simulink model "dynamic_range_compression"  (R2020b)
settings: Solver=FixedStepAuto  StartTime=0.0  StopTime=stop_time  FixedStep=1  RelTol=1e-3
InitFcn:
  | test_FFT_to_gain_init
StopFcn:
  | test_FFT_to_gain_stop
values from neighbouring files (symbols this model uses):
  accum_delay = max(band_sizes)    [test_FFT_to_gain_init.m]
  accum_delay_memory_size = 2^accum_delay_memory    [test_FFT_to_gain_init.m]
  band_edges = [band_edges mirrored_band_edges]    [test_FFT_to_gain_init.m]
  buf_a = 65.*ones(num_bands,1)    [test_FFT_to_gain_init.m]    (also in test_db_ar_gaintable_init.m)
  buf_r = 65.*ones(num_bands,1)    [test_FFT_to_gain_init.m]    (also in test_db_ar_gaintable_init.m)
  delay_memory_size = 2^system_delay_memory    [test_FFT_to_gain_init.m]
  FFTsize = 256    [test_FFT_to_gain_init.m]    (also in test_db_ar_gaintable_init.m)
  gainapp_dp_memory = log2(num_bands) + 1    [test_FFT_to_gain_init.m]
  num_bands = 8    [test_FFT_to_gain_init.m]    (also in test_db_ar_gaintable_init.m = 2)
  num_bins = FFTsize/2 + 1    (= 129)    [test_FFT_to_gain_init.m]    (also in test_db_ar_gaintable_init.m)
  system_delay = 70    [calculate_gainapp_test_signals.m]    (also in test_FFT_to_gain_init.m = gain_delay + accum_delay)
  table_length = length(gtdata)    [test_FFT_to_gain_init.m]    (also in test_db_ar_gaintable_init.m)
  X_high = 93    [test_FFT_to_gain_init.m]    (also in test_db_ar_gaintable_init.m)
undefined symbols (not defined in the file or in its folder): xIn
libraries: hdlsllib x8, simulink x8, FPGA_Open_Speech_Tools x5
(part 2 of 2)

== matlab function dynamic_range_compression/Gain Calculation/Intensity/Frequency Band Intensity Accumulator ==
  data: bin_intensity input; level_in output fixdt(1,Wbits,Fbits); accumulator_reset input; bin_num input; num_bins input
function level_in = accumulate_band(bin_intensity, accumulator_reset, bin_num, num_bins)

% Accumulates the bin intensities until a new frequency band is detected.
% Takes in the current frequency bin intensity, an accumulator reset
% control signal, bin number and number of frequency bins. If the 
% accumulator_reset is true, the sum is reset starting with the current 
% frequency bin intensity. Unless a DC or Nyquist bin is detected, a
% logical shift left is executed to apply a gain of two to the current
% bin_intensity, which accounts for negative frequencies.

persistent total;

if isempty(total)
    total = fi(0,1,40,32);
end

if bin_num == 0 || bin_num == num_bins-1
    dc_nyquist = true;
else
    dc_nyquist = false;
end

if accumulator_reset == true && dc_nyquist == true
    total = fi(bin_intensity,1,40,32);
    level_in = total;
elseif accumulator_reset == true && dc_nyquist == false
    total = bitsll(fi(bin_intensity,1,40,32),fi(1));
    level_in = total;
elseif accumulator_reset == false && dc_nyquist == true
    total = fi(total + fi(bin_intensity,1,40,32),1,40,32);
    level_in = total;
elseif accumulator_reset == false && dc_nyquist == false
    total = fi(total + bitsll(fi(bin_intensity,1,40,32),fi(1)),1,40,32);
    level_in = total;
else
    total = fi(0,1,40,32);
    error('Incorrect Logic in accumulate_band function!');
end
